simulink model "ARI_24_1_AW_Deadbeat"  (Simulink 7.8)
settings: Solver=ode45  StartTime=0.0  StopTime=6  RelTol=1e-3
values from neighbouring files (symbols this model uses):
  h = findobj(gcf,'type','line')    [boldLines.m]    (also in phase.m = min(hmax, 0.9*h*(tau/delta)^pow))
libraries: simulink x1
settings Model: Creator=Michael Sebek  ModifiedByFormat=Michael Sebek  LastModifiedBy=Michael Sebek
settings OptimizationCC: InitFltsAndDblsToZero=on
settings DebuggingCC: SaveWithParameterizedLinksMsg=none  SignalResolutionControl=TryResolveAllWithWarning  MultiTaskDSMMsg=warning  MultiTaskCondExecSysMsg=none  FcnCallInpInsideContextMsg=Use local settings  StrictBusMsg=None
settings RTWCC: IncludeERTFirstTime=on
settings GRTTargetCC: TargetFcnLib=ansi_tfl_tmw.mat

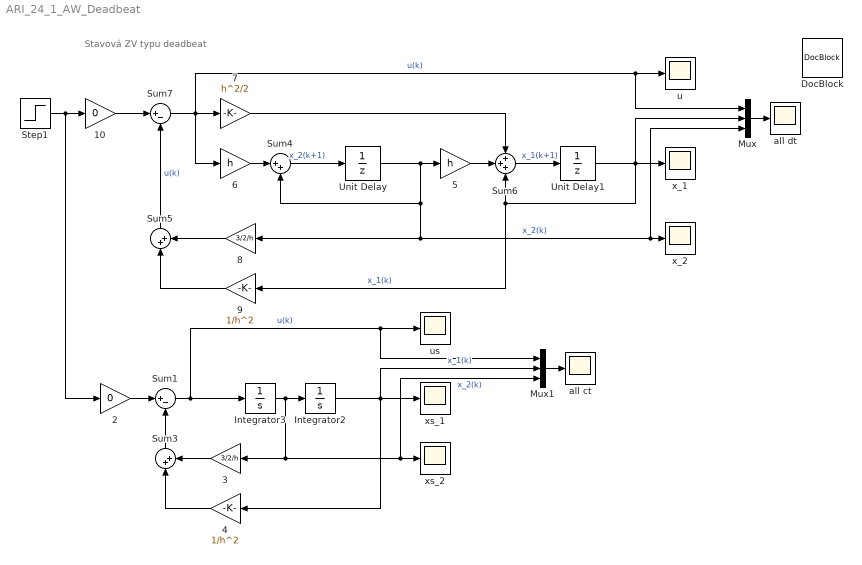
== system ARI_24_1_AW_Deadbeat ==
  note: Stavová ZV typu deadbeat
  10 : Gain  Gain=0  SampleTime=h
  2 : Gain  Gain=0
  3 : Gain  Gain=3/2/h  SampleTime=h
  4 : Gain  Gain=1/h^2  SampleTime=h
  5 : Gain  Gain=h  SampleTime=h
  6 : Gain  Gain=h  SampleTime=h
  7 : Gain  Gain=h^2/2  SampleTime=h
  8 : Gain  Gain=3/2/h  SampleTime=h
  9 : Gain  Gain=1/h^2  SampleTime=h
  DocBlock : simulink/Model-Wide Utilities/DocBlock  DocumentType=Text
      content=|
      | Sampling period must be defined:
      | h=1
  Integrator2 : Integrator  InitialCondition=1
  Integrator3 : Integrator  InitialCondition=1
  Mux : Mux  Inputs=3
  Mux1 : Mux  Inputs=3
  Step1 : Step  Time=0  SampleTime=0
  Sum1 : Sum  Inputs=|+-
  Sum3 : Sum  Inputs=|++
  Sum4 : Sum  Inputs=|++
  Sum5 : Sum  Inputs=|++
  Sum6 : Sum  Inputs=+++
  Sum7 : Sum  Inputs=|+-
  Unit Delay : UnitDelay  X0=1  SampleTime=h
  Unit Delay1 : UnitDelay  X0=1  SampleTime=h
  all ct : Scope
      settings: SaveName=ScopeData7
  all dt : Scope
      settings: SaveName=ScopeData6
  u : Scope
      settings: SaveName=ScopeData4
  us : Scope
      settings: TimeRange=6  YMin=-3  YMax=3  SaveName=ScopeData2
  x_1 : Scope
  x_2 : Scope
      settings: SaveName=ScopeData5
  xs_1 : Scope
      settings: SaveName=ScopeData3
  xs_2 : Scope
  wires:
  Integrator2/1 -> 4/1, xs_1/1, Mux1/2  "x_1(k)"
  Sum1/1 -> Integrator3/1, Mux1/1, us/1  "u(k)"
  2/1 -> Sum1/1
  Integrator3/1 -> Integrator2/1, 3/1, xs_2/1, Mux1/3  "x_2(k)"
  Sum3/1 -> Sum1/2
  4/1 -> Sum3/1
  3/1 -> Sum3/2
  Sum4/1 -> Unit Delay/1  "x_2(k+1)"
  Unit Delay/1 -> 5/1, Sum4/2, 8/1, x_2/1, Mux/3  "x_2(k)"
  Sum6/1 -> Unit Delay1/1  "x_1(k+1)"
  Unit Delay1/1 -> Sum6/3, 9/1, x_1/1, Mux/2  "x_1(k)"
  6/1 -> Sum4/1
  7/1 -> Sum6/1
  5/1 -> Sum6/2
  9/1 -> Sum5/1
  8/1 -> Sum5/2
  Sum7/1 -> 7/1, 6/1, u/1, Mux/1  "u(k)"
  Step1/1 -> 10/1, 2/1
  10/1 -> Sum7/1
  Sum5/1 -> Sum7/2  "u(k)"
  Mux/1 -> all dt/1
  Mux1/1 -> all ct/1
